simulink model "steeringsimulation"  (R2023b)
settings: Solver=VariableStepAuto  StartTime=0.0  StopTime=15  RelTol=1e-3
undefined symbols (not defined in the file): b_actual_ft, b_measured_ft, counts_to_rad, K_l, K_r, r_actual_ft, r_measured_ft, rad_to_counts, sigma_l, sigma_r, Ts, Unstable_V, V_max
libraries: slpidlib x4, simulink x2
settings Model: Creator=tvincent  LastModifiedBy=bensp
settings ModelReferenceCC: EnableRefExpFcnMdlSchedulingChecks=on

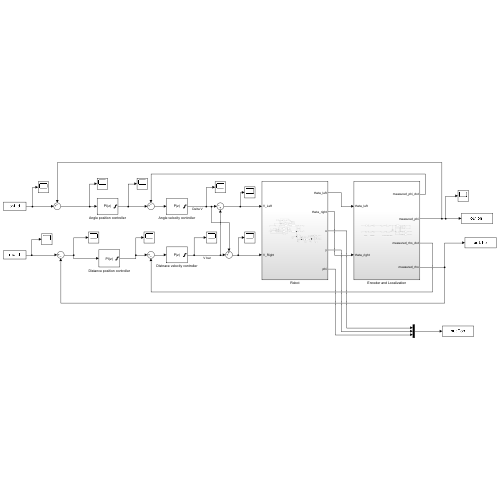
[thumbnail: Simulink's stored preview of the top-level diagram]
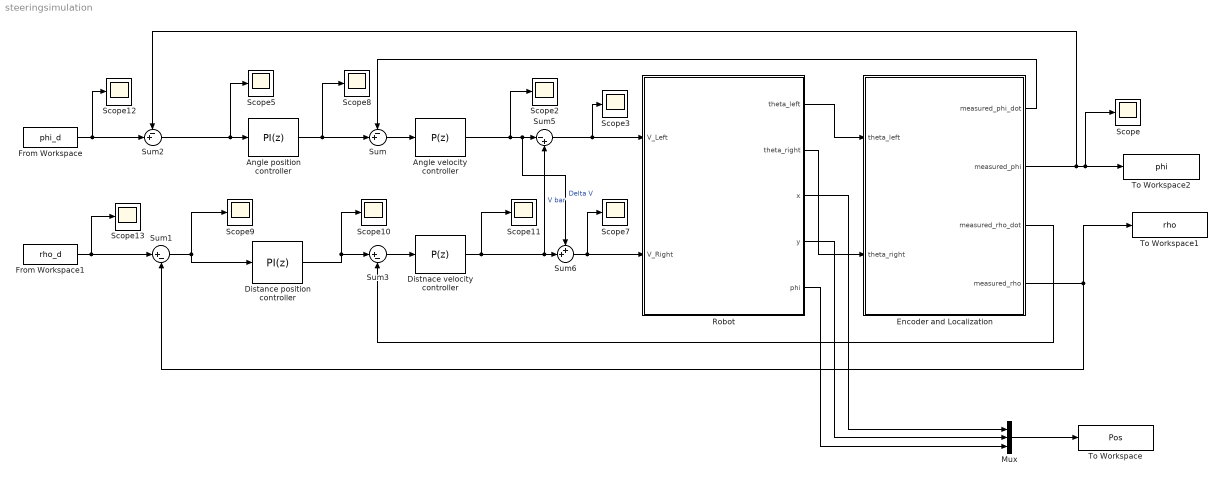
== system steeringsimulation ==
  Angle position controller : slpidlib/PID Controller  Controller=PI  Form=Parallel  TimeDomain=Discrete-time  UseExternalTs=off  SampleTime=Ts  IntegratorMethod=Forward Euler  FilterMethod=Forward Euler  ControllerParametersSource=internal  P=14.519508378545  I=38.3894759208685  UseKiTs=off  D=0.388544873825985  N=95.1837565933296  UseFilter=on  TunerSelectOption=Transfer Function Based (PID Tuner App)  InitialConditionSource=internal  InitialConditionForIntegrator=0  InitialConditionForFilter=0  DifferentiatorICPrevScaledInput=0  ExternalReset=none  TrackingMode=off  Kt=1  LimitOutput=on  SatLimitsSource=internal  UpperSaturationLimit=pi/2  LowerSaturationLimit=-pi/2  LinearizeAsGain=on  AntiWindupMode=clamping  Kb=1  LimitIntegrator=off  UpperIntegratorSaturationLimit=inf  LowerIntegratorSaturationLimit=-inf  POutMin=[]  POutMax=[]  IOutMin=[]  IOutMax=[]  DOutMin=[]  DOutMax=[]  NOutMin=[]  NOutMax=[]  SumOutMin=[]  SumOutMax=[]  SaturationOutMin=[]  SaturationOutMax=[]  PParamMin=[]  PParamMax=[]  IParamMin=[]  IParamMax=[]  DParamMin=[]  DParamMax=[]  NParamMin=[]  NParamMax=[]  KbParamMin=[]  KbParamMax=[]  KtParamMin=[]  KtParamMax=[]  KbOutMin=[]  KbOutMax=[]  KtOutMin=[]  KtOutMax=[]  IntegratorOutMin=[]  IntegratorOutMax=[]  FilterOutMin=[]  FilterOutMax=[]  SumI1OutMin=[]  SumI1OutMax=[]  SumI2OutMin=[]  SumI2OutMax=[]  SumI3OutMin=[]  SumI3OutMax=[]  SumI4OutMin=[]  SumI4OutMax=[]  SumDOutMin=[]  SumDOutMax=[]  DifferentiatorOutMin=[]  DifferentiatorOutMax=[]  FilterDiffOutCoefMin=[]  FilterDiffOutCoefMax=[]  ReciprocalOutMin=[]  ReciprocalOutMax=[]  SumDenOutMin=[]  SumDenOutMax=[]  SumNumOutMin=[]  SumNumOutMax=[]  DivideOutMin=[]  DivideOutMax=[]  UdiffTsProdOutMin=[]  UdiffTsProdOutMax=[]  NTsProdOutMin=[]  NTsProdOutMax=[]  UintegralTsProdOutMin=[]  UintegralTsProdOutMax=[]  UngainTsProdOutMin=[]  UngainTsProdOutMax=[]  ClampingZeroOutDataTypeStr=Inherit: Inherit via back propagation  ClampingZeroOutMin=[]  ClampingZeroOutMax=[]  FilterDenConstantOutDataTypeStr=Inherit: Inherit via back propagation  FilterDenConstantOutMin=[]  FilterDenConstantOutMax=[]  PCopyOutDataTypeStr=Inherit: Inherit via back propagation  PCopyOutMin=[]  PCopyOutMax=[]  NCopyOutDataTypeStr=Inherit: Inherit via back propagation  NCopyOutMin=[]  NCopyOutMax=[]  IntegratorContinuousStateAttributes=''  IntegratorStateMustResolveToSignalObject=off  IntegratorRTWStateStorageClass=Auto  FilterContinuousStateAttributes=''  FilterStateMustResolveToSignalObject=off  FilterRTWStateStorageClass=Auto  ParallelPVariant=InternalParameters  IdealPVariant=Disabled  IVariant=InternalParameters  DVariant=Disabled  IntegratorVariant=Discrete  SatVariant=Enabled  AWVariant=DiscClampingParallel  PCopyVariant=Disabled  TRVariant=Disabled  FdbkBlocksVariant=Forward  IdealPFdbkVariant=Disabled  SatFdbkVariant=Disabled  DerivativeFilterVariant=Disabled  NVariant=Disabled  NCopyVariant=Disabled_SignalSpec  FilterICVariant=Disabled  IntegratorICVariant=InternalICs  ExternalResetVariant=Disabled  TRSumVariant=Passthrough  SumFdbkVariant=Disabled  SumVariant=Sum_PI  TsampFilterVariant=InternalTs  TsampNgainVariant=Passthrough  TsampIntegralVariant=Disabled_SignalSpec  ExternalSaturationOutDataTypeStr=Inherit: Same as second input
  Angle velocity controller : slpidlib/PID Controller  Controller=P  Form=Parallel  TimeDomain=Discrete-time  UseExternalTs=off  SampleTime=-1  IntegratorMethod=Forward Euler  FilterMethod=Forward Euler  ControllerParametersSource=internal  P=6.80198490481403  I=0  UseKiTs=off  D=0  N=100  UseFilter=on  TunerSelectOption=Transfer Function Based (PID Tuner App)  InitialConditionSource=internal  InitialConditionForIntegrator=0  InitialConditionForFilter=0  DifferentiatorICPrevScaledInput=0  ExternalReset=none  TrackingMode=off  Kt=1  LimitOutput=on  SatLimitsSource=internal  UpperSaturationLimit=V_max  LowerSaturationLimit=-V_max  LinearizeAsGain=on  AntiWindupMode=none  Kb=1  LimitIntegrator=off  UpperIntegratorSaturationLimit=inf  LowerIntegratorSaturationLimit=-inf  POutMin=[]  POutMax=[]  IOutMin=[]  IOutMax=[]  DOutMin=[]  DOutMax=[]  NOutMin=[]  NOutMax=[]  SumOutMin=[]  SumOutMax=[]  SaturationOutMin=[]  SaturationOutMax=[]  PParamMin=[]  PParamMax=[]  IParamMin=[]  IParamMax=[]  DParamMin=[]  DParamMax=[]  NParamMin=[]  NParamMax=[]  KbParamMin=[]  KbParamMax=[]  KtParamMin=[]  KtParamMax=[]  KbOutMin=[]  KbOutMax=[]  KtOutMin=[]  KtOutMax=[]  IntegratorOutMin=[]  IntegratorOutMax=[]  FilterOutMin=[]  FilterOutMax=[]  SumI1OutMin=[]  SumI1OutMax=[]  SumI2OutMin=[]  SumI2OutMax=[]  SumI3OutMin=[]  SumI3OutMax=[]  SumI4OutMin=[]  SumI4OutMax=[]  SumDOutMin=[]  SumDOutMax=[]  DifferentiatorOutMin=[]  DifferentiatorOutMax=[]  FilterDiffOutCoefMin=[]  FilterDiffOutCoefMax=[]  ReciprocalOutMin=[]  ReciprocalOutMax=[]  SumDenOutMin=[]  SumDenOutMax=[]  SumNumOutMin=[]  SumNumOutMax=[]  DivideOutMin=[]  DivideOutMax=[]  UdiffTsProdOutMin=[]  UdiffTsProdOutMax=[]  NTsProdOutMin=[]  NTsProdOutMax=[]  UintegralTsProdOutMin=[]  UintegralTsProdOutMax=[]  UngainTsProdOutMin=[]  UngainTsProdOutMax=[]  ClampingZeroOutDataTypeStr=Inherit: Inherit via back propagation  ClampingZeroOutMin=[]  ClampingZeroOutMax=[]  FilterDenConstantOutDataTypeStr=Inherit: Inherit via back propagation  FilterDenConstantOutMin=[]  FilterDenConstantOutMax=[]  PCopyOutDataTypeStr=Inherit: Inherit via back propagation  PCopyOutMin=[]  PCopyOutMax=[]  NCopyOutDataTypeStr=Inherit: Inherit via back propagation  NCopyOutMin=[]  NCopyOutMax=[]  IntegratorContinuousStateAttributes=''  IntegratorStateMustResolveToSignalObject=off  IntegratorRTWStateStorageClass=Auto  FilterContinuousStateAttributes=''  FilterStateMustResolveToSignalObject=off  FilterRTWStateStorageClass=Auto  ParallelPVariant=InternalParameters  IdealPVariant=Disabled  IVariant=Disabled  DVariant=Disabled  IntegratorVariant=Disabled  SatVariant=Enabled  AWVariant=Disabled  PCopyVariant=Disabled  TRVariant=Disabled  FdbkBlocksVariant=Forward  IdealPFdbkVariant=Disabled  SatFdbkVariant=Disabled  DerivativeFilterVariant=Disabled  NVariant=Disabled  NCopyVariant=Disabled_SignalSpec  FilterICVariant=Disabled  IntegratorICVariant=Disabled  ExternalResetVariant=Disabled  TRSumVariant=Passthrough  SumFdbkVariant=Disabled  SumVariant=Passthrough_P  TsampFilterVariant=InternalTs  TsampNgainVariant=Passthrough  TsampIntegralVariant=Disabled_SignalSpec  ExternalSaturationOutDataTypeStr=Inherit: Same as second input
  Distance position controller : slpidlib/PID Controller  Controller=PI  Form=Parallel  TimeDomain=Discrete-time  UseExternalTs=off  SampleTime=Ts  IntegratorMethod=Forward Euler  FilterMethod=Forward Euler  ControllerParametersSource=internal  P=14.2423071458154  I=31.5620509245516  UseKiTs=off  D=0.388544873825985  N=95.1837565933296  UseFilter=on  TunerSelectOption=Transfer Function Based (PID Tuner App)  InitialConditionSource=internal  InitialConditionForIntegrator=0  InitialConditionForFilter=0  DifferentiatorICPrevScaledInput=0  ExternalReset=none  TrackingMode=off  Kt=1  LimitOutput=on  SatLimitsSource=internal  UpperSaturationLimit=0.5  LowerSaturationLimit=-0.5  LinearizeAsGain=on  AntiWindupMode=clamping  Kb=1  LimitIntegrator=off  UpperIntegratorSaturationLimit=inf  LowerIntegratorSaturationLimit=-inf  POutMin=[]  POutMax=[]  IOutMin=[]  IOutMax=[]  DOutMin=[]  DOutMax=[]  NOutMin=[]  NOutMax=[]  SumOutMin=[]  SumOutMax=[]  SaturationOutMin=[]  SaturationOutMax=[]  PParamMin=[]  PParamMax=[]  IParamMin=[]  IParamMax=[]  DParamMin=[]  DParamMax=[]  NParamMin=[]  NParamMax=[]  KbParamMin=[]  KbParamMax=[]  KtParamMin=[]  KtParamMax=[]  KbOutMin=[]  KbOutMax=[]  KtOutMin=[]  KtOutMax=[]  IntegratorOutMin=[]  IntegratorOutMax=[]  FilterOutMin=[]  FilterOutMax=[]  SumI1OutMin=[]  SumI1OutMax=[]  SumI2OutMin=[]  SumI2OutMax=[]  SumI3OutMin=[]  SumI3OutMax=[]  SumI4OutMin=[]  SumI4OutMax=[]  SumDOutMin=[]  SumDOutMax=[]  DifferentiatorOutMin=[]  DifferentiatorOutMax=[]  FilterDiffOutCoefMin=[]  FilterDiffOutCoefMax=[]  ReciprocalOutMin=[]  ReciprocalOutMax=[]  SumDenOutMin=[]  SumDenOutMax=[]  SumNumOutMin=[]  SumNumOutMax=[]  DivideOutMin=[]  DivideOutMax=[]  UdiffTsProdOutMin=[]  UdiffTsProdOutMax=[]  NTsProdOutMin=[]  NTsProdOutMax=[]  UintegralTsProdOutMin=[]  UintegralTsProdOutMax=[]  UngainTsProdOutMin=[]  UngainTsProdOutMax=[]  ClampingZeroOutDataTypeStr=Inherit: Inherit via back propagation  ClampingZeroOutMin=[]  ClampingZeroOutMax=[]  FilterDenConstantOutDataTypeStr=Inherit: Inherit via back propagation  FilterDenConstantOutMin=[]  FilterDenConstantOutMax=[]  PCopyOutDataTypeStr=Inherit: Inherit via back propagation  PCopyOutMin=[]  PCopyOutMax=[]  NCopyOutDataTypeStr=Inherit: Inherit via back propagation  NCopyOutMin=[]  NCopyOutMax=[]  IntegratorContinuousStateAttributes=''  IntegratorStateMustResolveToSignalObject=off  IntegratorRTWStateStorageClass=Auto  FilterContinuousStateAttributes=''  FilterStateMustResolveToSignalObject=off  FilterRTWStateStorageClass=Auto  ParallelPVariant=InternalParameters  IdealPVariant=Disabled  IVariant=InternalParameters  DVariant=Disabled  IntegratorVariant=Discrete  SatVariant=Enabled  AWVariant=DiscClampingParallel  PCopyVariant=Disabled  TRVariant=Disabled  FdbkBlocksVariant=Forward  IdealPFdbkVariant=Disabled  SatFdbkVariant=Disabled  DerivativeFilterVariant=Disabled  NVariant=Disabled  NCopyVariant=Disabled_SignalSpec  FilterICVariant=Disabled  IntegratorICVariant=InternalICs  ExternalResetVariant=Disabled  TRSumVariant=Passthrough  SumFdbkVariant=Disabled  SumVariant=Sum_PI  TsampFilterVariant=InternalTs  TsampNgainVariant=Passthrough  TsampIntegralVariant=Disabled_SignalSpec  ExternalSaturationOutDataTypeStr=Inherit: Same as second input
  Distnace velocity controller : slpidlib/PID Controller  Controller=P  Form=Parallel  TimeDomain=Discrete-time  UseExternalTs=off  SampleTime=-1  IntegratorMethod=Forward Euler  FilterMethod=Forward Euler  ControllerParametersSource=internal  P=10  I=1  UseKiTs=off  D=0  N=100  UseFilter=on  TunerSelectOption=Transfer Function Based (PID Tuner App)  InitialConditionSource=internal  InitialConditionForIntegrator=0  InitialConditionForFilter=0  DifferentiatorICPrevScaledInput=0  ExternalReset=none  TrackingMode=off  Kt=1  LimitOutput=on  SatLimitsSource=internal  UpperSaturationLimit=V_max  LowerSaturationLimit=-V_max  LinearizeAsGain=on  AntiWindupMode=none  Kb=1  LimitIntegrator=off  UpperIntegratorSaturationLimit=inf  LowerIntegratorSaturationLimit=-inf  POutMin=[]  POutMax=[]  IOutMin=[]  IOutMax=[]  DOutMin=[]  DOutMax=[]  NOutMin=[]  NOutMax=[]  SumOutMin=[]  SumOutMax=[]  SaturationOutMin=[]  SaturationOutMax=[]  PParamMin=[]  PParamMax=[]  IParamMin=[]  IParamMax=[]  DParamMin=[]  DParamMax=[]  NParamMin=[]  NParamMax=[]  KbParamMin=[]  KbParamMax=[]  KtParamMin=[]  KtParamMax=[]  KbOutMin=[]  KbOutMax=[]  KtOutMin=[]  KtOutMax=[]  IntegratorOutMin=[]  IntegratorOutMax=[]  FilterOutMin=[]  FilterOutMax=[]  SumI1OutMin=[]  SumI1OutMax=[]  SumI2OutMin=[]  SumI2OutMax=[]  SumI3OutMin=[]  SumI3OutMax=[]  SumI4OutMin=[]  SumI4OutMax=[]  SumDOutMin=[]  SumDOutMax=[]  DifferentiatorOutMin=[]  DifferentiatorOutMax=[]  FilterDiffOutCoefMin=[]  FilterDiffOutCoefMax=[]  ReciprocalOutMin=[]  ReciprocalOutMax=[]  SumDenOutMin=[]  SumDenOutMax=[]  SumNumOutMin=[]  SumNumOutMax=[]  DivideOutMin=[]  DivideOutMax=[]  UdiffTsProdOutMin=[]  UdiffTsProdOutMax=[]  NTsProdOutMin=[]  NTsProdOutMax=[]  UintegralTsProdOutMin=[]  UintegralTsProdOutMax=[]  UngainTsProdOutMin=[]  UngainTsProdOutMax=[]  ClampingZeroOutDataTypeStr=Inherit: Inherit via back propagation  ClampingZeroOutMin=[]  ClampingZeroOutMax=[]  FilterDenConstantOutDataTypeStr=Inherit: Inherit via back propagation  FilterDenConstantOutMin=[]  FilterDenConstantOutMax=[]  PCopyOutDataTypeStr=Inherit: Inherit via back propagation  PCopyOutMin=[]  PCopyOutMax=[]  NCopyOutDataTypeStr=Inherit: Inherit via back propagation  NCopyOutMin=[]  NCopyOutMax=[]  IntegratorContinuousStateAttributes=''  IntegratorStateMustResolveToSignalObject=off  IntegratorRTWStateStorageClass=Auto  FilterContinuousStateAttributes=''  FilterStateMustResolveToSignalObject=off  FilterRTWStateStorageClass=Auto  ParallelPVariant=InternalParameters  IdealPVariant=Disabled  IVariant=Disabled  DVariant=Disabled  IntegratorVariant=Disabled  SatVariant=Enabled  AWVariant=Disabled  PCopyVariant=Disabled  TRVariant=Disabled  FdbkBlocksVariant=Forward  IdealPFdbkVariant=Disabled  SatFdbkVariant=Disabled  DerivativeFilterVariant=Disabled  NVariant=Disabled  NCopyVariant=Disabled_SignalSpec  FilterICVariant=Disabled  IntegratorICVariant=Disabled  ExternalResetVariant=Disabled  TRSumVariant=Passthrough  SumFdbkVariant=Disabled  SumVariant=Passthrough_P  TsampFilterVariant=InternalTs  TsampNgainVariant=Passthrough  TsampIntegralVariant=Disabled_SignalSpec  ExternalSaturationOutDataTypeStr=Inherit: Same as second input
  Encoder and Localization : Subsystem
  From Workspace : FromWorkspace  VariableName=phi_d
  From Workspace1 : FromWorkspace  VariableName=rho_d
  Mux : Mux  Inputs=3
  Robot : Subsystem
  Scope{,2..3,5,7..13} (11 alike) : Scope
  Sum : Sum  Inputs=-+|
  Sum1 : Sum  Inputs=|+-
  Sum2 : Sum  Inputs=-+|
  Sum3 : Sum  Inputs=|+-
  Sum5 : Sum  Inputs=|-+
  Sum6 : Sum  Inputs=++|
  To Workspace : ToWorkspace  VariableName=Pos  SaveFormat=Timeseries  SampleTime=.1
  To Workspace1 : ToWorkspace  VariableName=rho  SaveFormat=Timeseries  SampleTime=.1
  To Workspace2 : ToWorkspace  VariableName=phi  SaveFormat=Timeseries  SampleTime=.1
  wires:
  Sum/1 -> Angle velocity controller/1
  Angle position controller/1 -> Scope8/1, Sum/2
  From Workspace1/1 -> Scope13/1, Sum1/1
  From Workspace/1 -> Scope12/1, Sum2/2
  Sum6/1 -> Robot/2(V_Right), Scope7/1
  Sum5/1 -> Robot/1(V_Left), Scope3/1
  Robot/1(theta_left) -> Encoder and Localization/1(theta_left)
  Encoder and Localization/3(measured_rho_dot) -> Sum3/2
  Encoder and Localization/1(measured_phi_dot) -> Sum/1
  Encoder and Localization/2(measured_phi) -> Scope/1, To Workspace2/1, Sum2/1
  Distnace velocity controller/1 -> Scope11/1, Sum5/2, Sum6/2  "V bar"
  Sum2/1 -> Scope5/1, Angle position controller/1
  Angle velocity controller/1 -> Scope2/1, Sum6/1, Sum5/1  "Delta V"
  Sum3/1 -> Distnace velocity controller/1
  Distance position controller/1 -> Scope10/1, Sum3/1
  Sum1/1 -> Scope9/1, Distance position controller/1
  Robot/4(y) -> Mux/2
  Robot/5(phi) -> Mux/3
  Robot/2(theta_right) -> Encoder and Localization/2(theta_right)
  Robot/3(x) -> Mux/1
  Mux/1 -> To Workspace/1
  Encoder and Localization/4(measured_rho) -> To Workspace1/1, Sum1/2

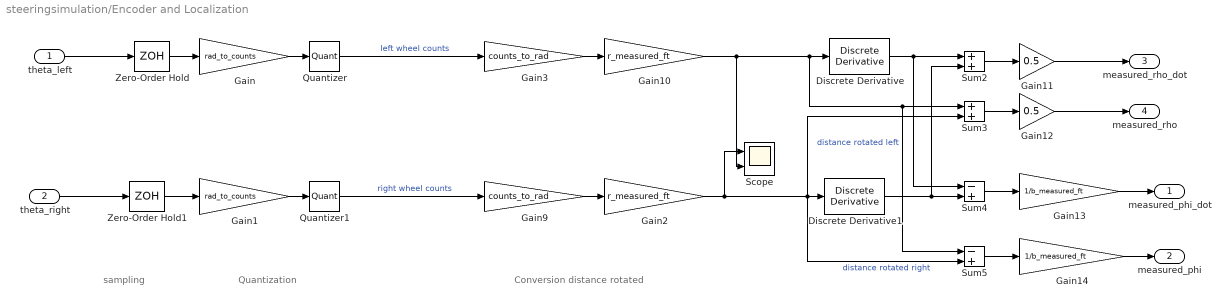
== system steeringsimulation/Encoder and Localization ==
  note: sampling
  note: Quantization
  note: Conversion distance rotated
  theta_left : Inport
  theta_right : Inport  Port=2
  Discrete Derivative : simulink/Discrete/Discrete Derivative  gainval=1  ICPrevScaledInput=0.0  OutMin=[]  OutMax=[]  OutDataType=fixdt(1, 16)  OutScaling=2^-10  DoSatur=off
  Discrete Derivative1 : simulink/Discrete/Discrete Derivative  gainval=1  ICPrevScaledInput=0.0  OutMin=[]  OutMax=[]  OutDataType=fixdt(1, 16)  OutScaling=2^-10  DoSatur=off
  Gain : Gain  Gain=rad_to_counts
  Gain1 : Gain  Gain=rad_to_counts
  Gain10 : Gain  Gain=r_measured_ft
  Gain11 : Gain  Gain=0.5
  Gain12 : Gain  Gain=0.5
  Gain13 : Gain  Gain=1/b_measured_ft
  Gain14 : Gain  Gain=1/b_measured_ft
  Gain2 : Gain  Gain=r_measured_ft
  Gain3 : Gain  Gain=counts_to_rad
  Gain9 : Gain  Gain=counts_to_rad
  Quantizer : Quantizer  QuantizationInterval=1
  Quantizer1 : Quantizer  QuantizationInterval=1
  Scope : Scope  NumInputPorts=2
  Sum2 : Sum
  Sum3 : Sum
  Sum4 : Sum  Inputs=-+
  Sum5 : Sum  Inputs=-+
  Zero-Order Hold : ZeroOrderHold  SampleTime=Ts
  Zero-Order Hold1 : ZeroOrderHold  SampleTime=Ts
  measured_phi_dot : Outport
  measured_phi : Outport  Port=2
  measured_rho_dot : Outport  Port=3
  measured_rho : Outport  Port=4
  wires:
  Zero-Order Hold/1 -> Gain/1
  Discrete Derivative/1 -> Sum4/1, Sum2/1
  Gain/1 -> Quantizer/1
  Quantizer/1 -> Gain3/1  "left wheel counts"
  Gain3/1 -> Gain10/1
  Gain10/1 -> Scope/2, Sum5/1, Sum3/1, Discrete Derivative/1  "distance rotated left"
  Quantizer1/1 -> Gain9/1  "right wheel counts"
  Gain9/1 -> Gain2/1
  Discrete Derivative1/1 -> Sum4/2, Sum2/2
  Zero-Order Hold1/1 -> Gain1/1
  Gain1/1 -> Quantizer1/1
  Gain2/1 -> Sum5/2, Discrete Derivative1/1, Sum3/2, Scope/1  "distance rotated right"
  Sum2/1 -> Gain11/1
  Gain11/1 -> measured_rho_dot/1
  Sum3/1 -> Gain12/1
  Gain12/1 -> measured_rho/1
  Gain13/1 -> measured_phi_dot/1
  Sum4/1 -> Gain13/1
  Gain14/1 -> measured_phi/1
  Sum5/1 -> Gain14/1
  theta_left/1 -> Zero-Order Hold/1
  theta_right/1 -> Zero-Order Hold1/1

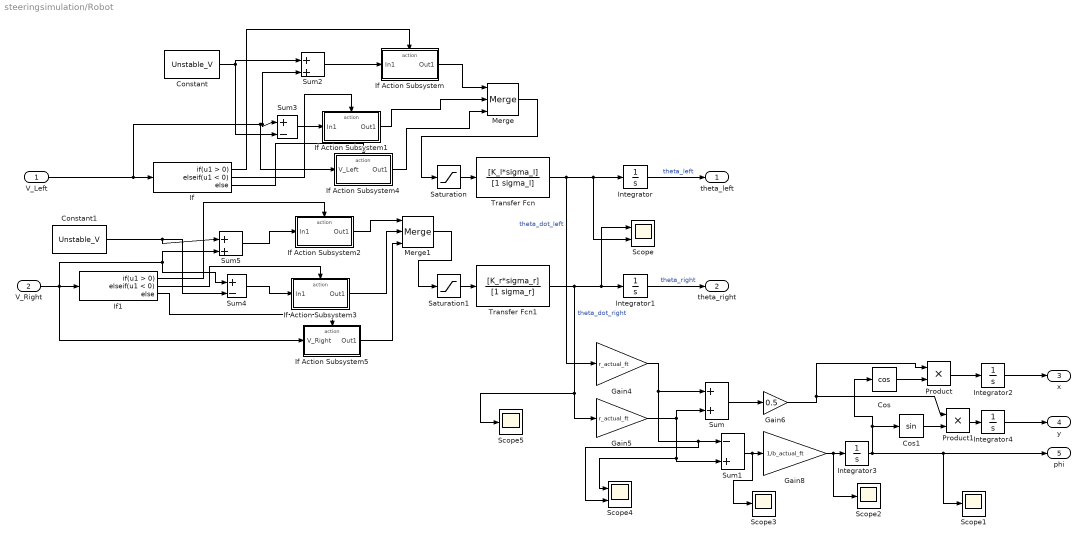
== system steeringsimulation/Robot ==
  V_Left : Inport
  V_Right : Inport  Port=2
  Constant : Constant  Value=Unstable_V
  Constant1 : Constant  Value=Unstable_V
  Cos : Trigonometry  Operator=cos
  Cos1 : Trigonometry
  Gain4 : Gain  Gain=r_actual_ft
  Gain5 : Gain  Gain=r_actual_ft
  Gain6 : Gain  Gain=0.5
  Gain8 : Gain  Gain=1/b_actual_ft
  If : If  ElseIfExpressions=u1 < 0
  If Action Subsystem : Subsystem  TreatAsAtomicUnit=on
  If Action Subsystem1 : Subsystem  TreatAsAtomicUnit=on
  If Action Subsystem2 : Subsystem  TreatAsAtomicUnit=on
  If Action Subsystem3 : Subsystem  TreatAsAtomicUnit=on
  If Action Subsystem4 : Subsystem  TreatAsAtomicUnit=on
  If Action Subsystem5 : Subsystem  TreatAsAtomicUnit=on
  If1 : If  ElseIfExpressions=u1 < 0
  Integrator{,1..4} (5 alike) : Integrator
  Merge : Merge  Inputs=3
  Merge1 : Merge  Inputs=3
  Product : Product
  Product1 : Product
  Saturation : Saturate  UpperLimit=V_max  LowerLimit=-V_max
  Saturation1 : Saturate  UpperLimit=V_max+Unstable_V  LowerLimit=-(V_max+Unstable_V)
  Scope : Scope  NumInputPorts=2
  Scope{1..3,5} (4 alike) : Scope
  Scope4 : Scope  NumInputPorts=2
  Sum : Sum
  Sum1 : Sum  Inputs=-+
  Sum2 : Sum  Inputs=|++
  Sum3 : Sum  Inputs=|+-
  Sum4 : Sum  Inputs=|+-
  Sum5 : Sum  Inputs=|++
  Transfer Fcn : TransferFcn  Numerator=[K_l*sigma_l]  Denominator=[1 sigma_l]
  Transfer Fcn1 : TransferFcn  Numerator=[K_r*sigma_r]  Denominator=[1 sigma_r]
  theta_left : Outport
  theta_right : Outport  Port=2
  x : Outport  Port=3
  y : Outport  Port=4
  phi : Outport  Port=5
  wires:
  Transfer Fcn/1 -> Gain4/1, Scope/2, Integrator/1  "theta_dot_left"
  Saturation/1 -> Transfer Fcn/1
  V_Right/1 -> If Action Subsystem5/1(V_Right), Sum5/2, Sum4/1, If1/1
  Saturation1/1 -> Transfer Fcn1/1
  Transfer Fcn1/1 -> Scope5/1, Gain5/1, Scope/1, Integrator1/1  "theta_dot_right"
  Sum/1 -> Gain6/1
  Integrator2/1 -> x/1
  Gain5/1 -> Sum/2, Scope4/1, Sum1/2
  Sum1/1 -> Scope3/1, Gain8/1
  Gain4/1 -> Scope4/2, Sum1/1, Sum/1
  Integrator3/1 -> Scope1/1, phi/1, Cos1/1, Cos/1
  Gain8/1 -> Scope2/1, Integrator3/1
  Gain6/1 -> Product1/1, Product/1
  Product/1 -> Integrator2/1
  Cos/1 -> Product/2
  Cos1/1 -> Product1/2
  Product1/1 -> Integrator4/1
  Integrator4/1 -> y/1
  Integrator/1 -> theta_left/1  "theta_left"
  Integrator1/1 -> theta_right/1  "theta_right"
  V_Left/1 -> If Action Subsystem4/1(V_Left), Sum3/1, Sum2/2, If/1
  Constant/1 -> Sum3/2, Sum2/1
  If/1 -> If Action Subsystem/Action
  Sum2/1 -> If Action Subsystem/1(In1)
  If Action Subsystem/1(Out1) -> Merge/1
  Merge/1 -> Saturation/1
  Sum3/1 -> If Action Subsystem1/1(In1)
  If Action Subsystem1/1(Out1) -> Merge/2
  If/2 -> If Action Subsystem1/Action
  Constant1/1 -> Sum4/2, Sum5/1
  If1/1 -> If Action Subsystem2/Action
  Sum5/1 -> If Action Subsystem2/1(In1)
  If Action Subsystem2/1(Out1) -> Merge1/1
  If1/2 -> If Action Subsystem3/Action
  Sum4/1 -> If Action Subsystem3/1(In1)
  If Action Subsystem3/1(Out1) -> Merge1/2
  Merge1/1 -> Saturation1/1
  If/3 -> If Action Subsystem4/Action
  If Action Subsystem4/1(Out1) -> Merge/3
  If1/3 -> If Action Subsystem5/Action
  If Action Subsystem5/1(Out1) -> Merge1/3

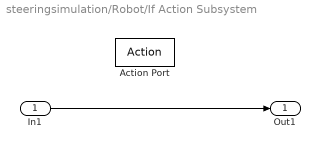
== system steeringsimulation/Robot/If Action Subsystem ==
  In1 : Inport
  Action Port : ActionPort  ActionPortLabel=if(u1 > 0)
  Out1 : Outport
  wires:
  In1/1 -> Out1/1

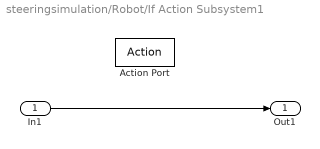
== system steeringsimulation/Robot/If Action Subsystem1 ==
  In1 : Inport
  Action Port : ActionPort  ActionPortLabel=elseif(u1 < 0)
  Out1 : Outport
  wires:
  In1/1 -> Out1/1

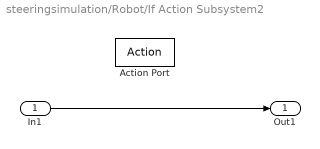
== system steeringsimulation/Robot/If Action Subsystem2 ==
  In1 : Inport
  Action Port : ActionPort  ActionPortLabel=if(u1 > 0)
  Out1 : Outport
  wires:
  In1/1 -> Out1/1

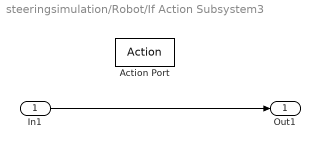
== system steeringsimulation/Robot/If Action Subsystem3 ==
  In1 : Inport
  Action Port : ActionPort  ActionPortLabel=elseif(u1 < 0)
  Out1 : Outport
  wires:
  In1/1 -> Out1/1

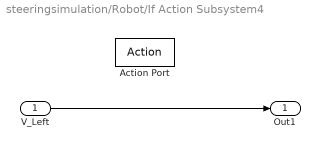
== system steeringsimulation/Robot/If Action Subsystem4 ==
  V_Left : Inport
  Action Port : ActionPort  ActionPortLabel=else
  Out1 : Outport
  wires:
  V_Left/1 -> Out1/1

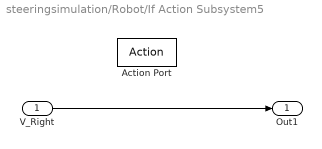
== system steeringsimulation/Robot/If Action Subsystem5 ==
  V_Right : Inport
  Action Port : ActionPort  ActionPortLabel=else
  Out1 : Outport
  wires:
  V_Right/1 -> Out1/1
